simulink model "homework6_model"  (R2013a)
settings: Solver=ode45  StartTime=0.0  StopTime=20  RelTol=1e-3
undefined symbols (not defined in the file or in its folder): pd
libraries: simulink x1
settings Model: Creator=wyh716  LastModifiedBy=wyh716

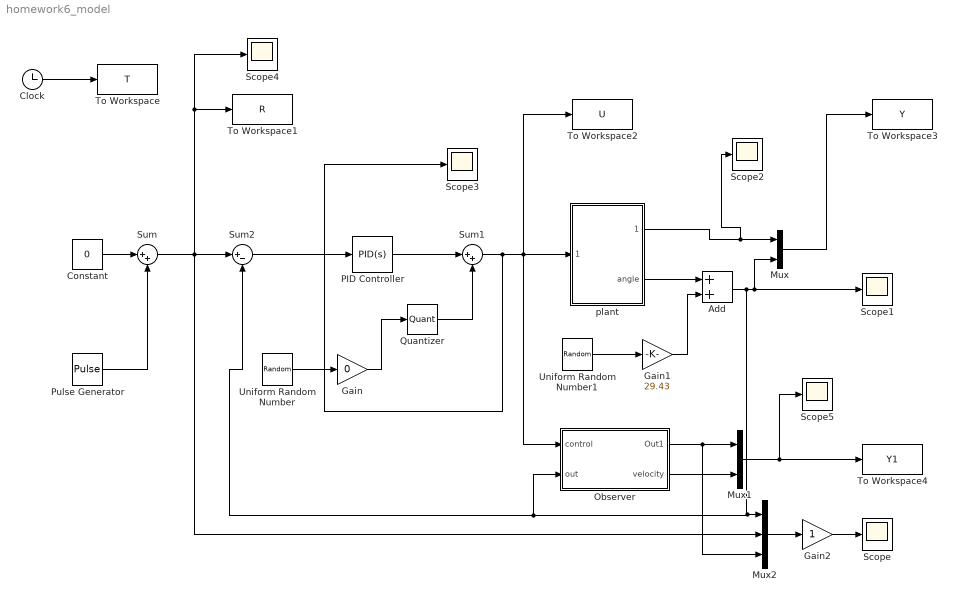
== system homework6_model ==
  Add : Sum
  Clock : Clock
  Constant : Constant  Value=0
  Gain : Gain  Gain=0
  Gain1 : Gain  Gain=29.43
  Gain2 : Gain
  Mux : Mux  Inputs=2
  Mux1 : Mux  Inputs=2
  Mux2 : Mux  Inputs=3
  Observer : Subsystem
  PID Controller : simulink/Continuous/PID Controller  Controller=PID  TimeDomain=Continuous-time  SampleTime=1  IntegratorMethod=Forward Euler  FilterMethod=Forward Euler  Form=Parallel  P=1.3429  I=2.6944  D=0.16398  N=130  InitialConditionSource=internal  InitialConditionForIntegrator=0  InitialConditionForFilter=0  ExternalReset=none  LimitOutput=off  UpperSaturationLimit=inf  LowerSaturationLimit=-inf  LinearizeAsGain=on  AntiWindupMode=none  Kb=1  TrackingMode=off  Kt=1  PParamMin=[]  PParamMax=[]  IParamMin=[]  IParamMax=[]  DParamMin=[]  DParamMax=[]  NParamMin=[]  NParamMax=[]  KbParamMin=[]  KbParamMax=[]  KtParamMin=[]  KtParamMax=[]  POutMin=[]  POutMax=[]  IOutMin=[]  IOutMax=[]  DOutMin=[]  DOutMax=[]  NOutMin=[]  NOutMax=[]  KbOutMin=[]  KbOutMax=[]  KtOutMin=[]  KtOutMax=[]  IntegratorOutMin=[]  IntegratorOutMax=[]  FilterOutMin=[]  FilterOutMax=[]  SumOutMin=[]  SumOutMax=[]  SumI1OutMin=[]  SumI1OutMax=[]  SumI2OutMin=[]  SumI2OutMax=[]  SumI3OutMin=[]  SumI3OutMax=[]  SumDOutMin=[]  SumDOutMax=[]  SaturationOutMin=[]  SaturationOutMax=[]  IntegratorContinuousStateAttributes=''  IntegratorStateMustResolveToSignalObject=off  IntegratorRTWStateStorageClass=Auto  FilterContinuousStateAttributes=''  FilterStateMustResolveToSignalObject=off  FilterRTWStateStorageClass=Auto
  Pulse Generator : DiscretePulseGenerator  PulseType=Time based  Amplitude=0.02  Period=0.1  PulseWidth=50  SampleTime=0.01
  Quantizer : Quantizer
  Scope{,1..5} (6 alike) : Scope
      Scope2 settings: SaveName=ScopeData2
      Scope3 settings: SaveName=ScopeData3
      Scope4 settings: SaveName=ScopeData4
      Scope5 settings: SaveName=ScopeData5
  Sum : Sum  Inputs=|++
  Sum1 : Sum  Inputs=|++
  Sum2 : Sum  Inputs=|+-
  To Workspace : ToWorkspace  VariableName=T  SampleTime=-1  SaveFormat=Timeseries
  To Workspace1 : ToWorkspace  VariableName=R  SampleTime=-1  SaveFormat=Timeseries
  To Workspace2 : ToWorkspace  VariableName=U  SampleTime=-1  SaveFormat=Timeseries
  To Workspace3 : ToWorkspace  VariableName=Y  SampleTime=-1  SaveFormat=Timeseries
  To Workspace4 : ToWorkspace  VariableName=Y1  SampleTime=-1  SaveFormat=Timeseries
  Uniform Random Number : UniformRandomNumber  SampleTime=0.01
  Uniform Random Number1 : UniformRandomNumber  SampleTime=0.1
  plant : Subsystem
  wires:
  Clock/1 -> To Workspace/1
  Sum/1 -> Sum2/1, Mux2/2, Scope4/1, To Workspace1/1
  Uniform Random Number/1 -> Gain/1
  Gain/1 -> Quantizer/1
  Quantizer/1 -> Sum1/2
  Sum1/1 -> Scope3/1, Observer/1(control), To Workspace2/1, plant/1(control)
  Uniform Random Number1/1 -> Gain1/1
  Gain1/1 -> Add/2
  plant/2(angle) -> Add/1
  Add/1 -> Sum2/2, Observer/2(out), Mux2/1, Mux/2, Scope1/1
  plant/1(velocity) -> Scope2/1, Mux/1
  Mux/1 -> To Workspace3/1
  Observer/1(Out1) -> Mux2/3, Mux1/1
  Observer/2(velocity) -> Mux1/2
  Mux1/1 -> Scope5/1, To Workspace4/1
  Mux2/1 -> Gain2/1
  Gain2/1 -> Scope/1
  PID Controller/1 -> Sum1/1
  Sum2/1 -> PID Controller/1
  Constant/1 -> Sum/1
  Pulse Generator/1 -> Sum/2

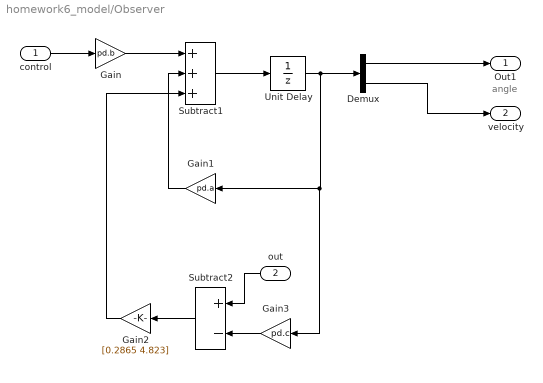
== system homework6_model/Observer ==
  note: angle
  control : Inport
  out : Inport  Port=2
  Demux : Demux  Outputs=2
  Gain : Gain  Gain=pd.b
  Gain1 : Gain  Gain=pd.a
  Gain2 : Gain  Gain=[0.2865 4.823]
  Gain3 : Gain  Gain=pd.c
  Subtract1 : Sum  Inputs=+++
  Subtract2 : Sum  Inputs=+-
  Unit Delay : UnitDelay  SampleTime=-1
  Out1 : Outport
  velocity : Outport  Port=2
  wires:
  control/1 -> Gain/1
  Gain/1 -> Subtract1/1
  Subtract1/1 -> Unit Delay/1
  Unit Delay/1 -> Gain3/1, Gain1/1, Demux/1
  Demux/1 -> Out1/1
  Demux/2 -> velocity/1
  out/1 -> Subtract2/1
  Gain3/1 -> Subtract2/2
  Subtract2/1 -> Gain2/1
  Gain2/1 -> Subtract1/3
  Gain1/1 -> Subtract1/2

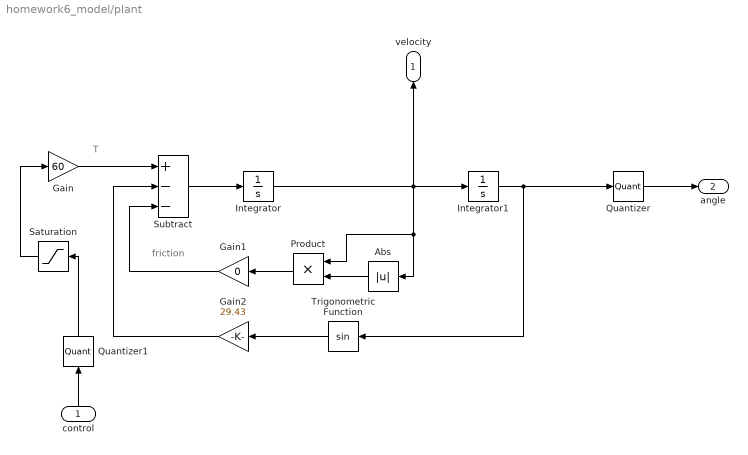
== system homework6_model/plant ==
  note: T
  note: friction
  control : Inport
  Abs : Abs
  Gain : Gain  Gain=60
  Gain1 : Gain  Gain=0
  Gain2 : Gain  Gain=29.43
  Integrator : Integrator
  Integrator1 : Integrator
  Product : Product
  Quantizer : Quantizer
  Quantizer1 : Quantizer
  Saturation : Saturate
  Subtract : Sum  Inputs=+--
  Trigonometric Function : Trigonometry
  velocity : Outport
  angle : Outport  Port=2
  wires:
  control/1 -> Quantizer1/1
  Quantizer1/1 -> Saturation/1
  Saturation/1 -> Gain/1
  Gain/1 -> Subtract/1
  Trigonometric Function/1 -> Gain2/1
  Product/1 -> Gain1/1
  Gain2/1 -> Subtract/2
  Gain1/1 -> Subtract/3
  Abs/1 -> Product/2
  Subtract/1 -> Integrator/1
  Integrator/1 -> Integrator1/1, Abs/1, Product/1, velocity/1
  Integrator1/1 -> Quantizer/1, Trigonometric Function/1
  Quantizer/1 -> angle/1
